simulink model "fullPlant"  (R2019a)
settings: Solver=VariableStepAuto  StartTime=0.0  StopTime=10.0  RelTol=1e-3
values from neighbouring files (symbols this model uses):
  alpha0 = 2    [aeroData.mat]
  b = 4.33    [aeroData.mat]
  c = 0.636    [aeroData.mat]
  CD = [0.01 0.012 0.015 0.019 0.024 0.03 0.036 0.044 0.052 0.01 0.012 0.015 ... (27 elements, 9x3)]    [aeroData.mat]
  Cl = [0.00012 -0.000325 -0.000768 -0.00121 -0.00165 -0.00209 -0.002529 -0.002968 -0.003408 -0.003849 -0.004292 0.002212 ... (33 elements, 11x3)]    [aeroData.mat]
  CL = [0.251 0.336 0.421 0.506 0.591 0.675 0.759 0.842 0.925 0.239 0.325 0.41 ... (27 elements, 9x3)]    [aeroData.mat]
  Clp = -0.00816971169566    [aeroData.mat]
  Clr = 0.00184411488766    [aeroData.mat]
  Cm = [-0.024 -0.038 -0.053 -0.068 -0.083 -0.098 -0.113 -0.128 -0.143 0.009 -0.005 -0.019 ... (27 elements, 9x3)]    [aeroData.mat]
  Cmq = -0.156184278773    [aeroData.mat]
  Cn = [-0.003061 -0.000518 0.002031 0.004586 0.007141 0.009696 0.012246 0.01479 0.017324 0.019845 0.022352 -0.012727 ... (33 elements, 11x3)]    [aeroData.mat]
  Cnp = -0.000739408737607    [aeroData.mat]
  Cnr = -0.00225688525575    [aeroData.mat]
  CY = [0.007395 0.001575 -0.004243 -0.010063 -0.015881 -0.021696 -0.027509 -0.033318 -0.039118 -0.044916 -0.050714 0.029115 ... (33 elements, 11x3)]    [aeroData.mat]
  g = 9.81    [aeroData.mat]
  gamma0 = -2.8361410859    [aeroData.mat]
  Ixx = 5.6481    [aeroData.mat]
  Iyy = 6.01051    [aeroData.mat]
  Izz = 11.4233    [aeroData.mat]
  m = 38    [aeroData.mat]
  S = 2.678    [aeroData.mat]
  V0 = 27    [aeroData.mat]
libraries: simulink x4, simulink_extras x3, aerolib6dof2 x1, aerolibatmos2 x1, aerolibasang x1, aerolibtransform2 x1, sharedtransform x1
settings Model: Creator=Admin  LastModifiedBy=Admin

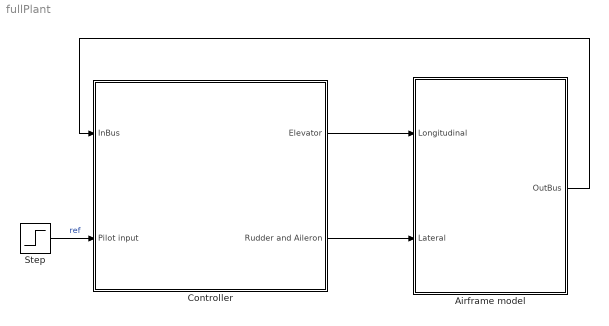
== system fullPlant ==
  Airframe model : Subsystem
  Controller : Subsystem
  Step : Step  Time=5  SampleTime=0
  wires:
  Step/1 -> Controller/2(Pilot input)  "ref"
  Controller/1(Elevator) -> Airframe model/1(Longitudinal)
  Controller/2(Rudder and Aileron) -> Airframe model/2(Lateral)
  Airframe model/1(OutBus) -> Controller/1(InBus)

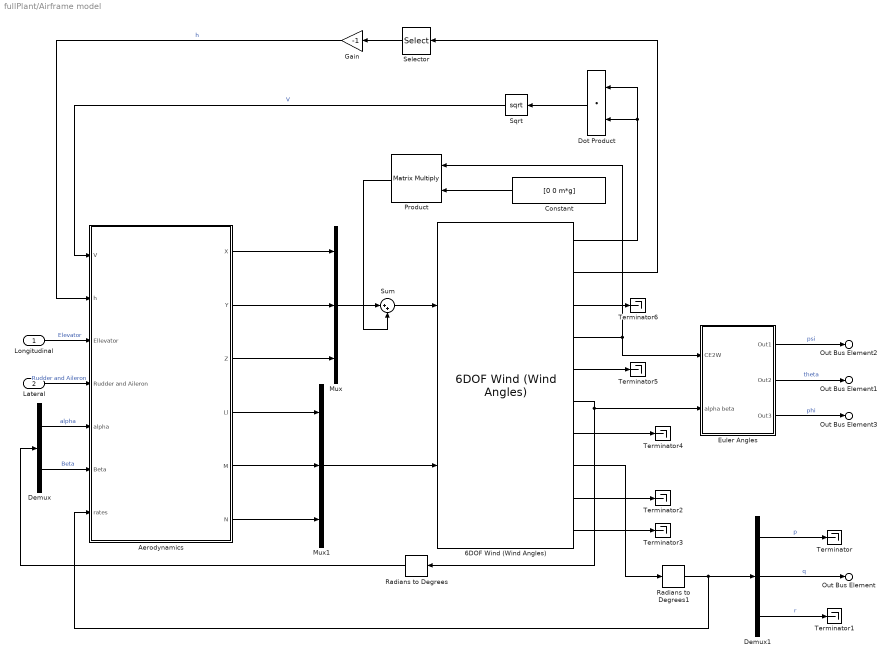
== system fullPlant/Airframe model ==
  Longitudinal : Inport
  Lateral : Inport  Port=2
  6DOF Wind (Wind Angles) : aerolib6dof2/6DOF Wind (Wind Angles)  units=Metric (MKS)  mtype=Fixed  rep=Wind Angles  xme_0=[0 0 -1000]  Vm_0=[V0 deg2rad(alpha0) 0]  wind_0=[0 deg2rad(gamma0) 0]  pm_0=[0 0 0]  mass_0=m  mass_e=0.5  mass_f=2.0  inertia=diag([Ixx Iyy Izz])  inertia_e=eye(3)  inertia_f=2*eye(3)  vre_flag=on  abi_flag=off  xme_statename=''  Vm_statename=''  alpha_statename=''  beta_statename=''  wind_statename=''  quat_statename=''  pm_statename=''  mass_statename=''
      settings: SourceProductName=Aerospace Blockset  SourceProductBaseCode=AE
  Aerodynamics : Subsystem
  Constant : Constant  Value=[0 0 m*g]
  Demux : Demux  Outputs=2
  Demux1 : Demux  Outputs=3
  Dot Product : DotProduct  InputSameDT=on  OutDataTypeStr=Inherit: Inherit via internal rule
  Euler Angles : Subsystem
  Gain : Gain  Gain=-1
  Mux : Mux  Inputs=3
  Mux1 : Mux  Inputs=3
  Product : Product  Multiplication=Matrix(*)
  Radians to Degrees : simulink_extras/Transformations/Radians to Degrees
  Radians to Degrees1 : simulink_extras/Transformations/Radians to Degrees
  Selector : Selector  InputPortWidth=3  IndexOptions=Index vector (dialog)  Indices=3  OutputSizes=1
  Sqrt : Sqrt  SaturateOnIntegerOverflow=on
  Sum : Sum  Inputs=|++
  Terminator{,1..6} (7 alike) : Terminator
  Out Bus Element : Outport  PortName=OutBus  Element=q
  Out Bus Element1 : Outport  PortName=OutBus  Element=theta
  Out Bus Element2 : Outport  PortName=OutBus  Element=psi
  Out Bus Element3 : Outport  PortName=OutBus  Element=phi
  wires:
  6DOF Wind (Wind Angles)/5 -> Terminator5/1
  Demux1/2 -> Out Bus Element/1  "q"
  Aerodynamics/4(Ll) -> Mux1/1
  Longitudinal/1 -> Aerodynamics/3(Ellevator)  "Elevator"
  Demux1/3 -> Terminator1/1  "r"
  6DOF Wind (Wind Angles)/4 -> Euler Angles/1(CE2W), Product/1
  Aerodynamics/5(M) -> Mux1/2
  6DOF Wind (Wind Angles)/9 -> Terminator2/1
  6DOF Wind (Wind Angles)/6 -> Radians to Degrees/1, Euler Angles/2(alpha beta)
  6DOF Wind (Wind Angles)/2 -> Selector/1
  6DOF Wind (Wind Angles)/10 -> Terminator3/1
  Lateral/1 -> Aerodynamics/4(Rudder and Aileron)  "Rudder and Aileron"
  Aerodynamics/3(Z) -> Mux/3
  Euler Angles/1(Out1) -> Out Bus Element2/1  "psi"
  6DOF Wind (Wind Angles)/1 -> Dot Product/1, Dot Product/2
  Aerodynamics/2(Y) -> Mux/2
  Demux/2 -> Aerodynamics/6(Beta)  "Beta"
  Sqrt/1 -> Aerodynamics/1(V)  "V"
  Dot Product/1 -> Sqrt/1
  Product/1 -> Sum/2
  6DOF Wind (Wind Angles)/3 -> Terminator6/1
  6DOF Wind (Wind Angles)/7 -> Terminator4/1
  Gain/1 -> Aerodynamics/2(h)  "h"
  Radians to Degrees/1 -> Demux/1
  Mux1/1 -> 6DOF Wind (Wind Angles)/2
  Aerodynamics/1(X) -> Mux/1
  Selector/1 -> Gain/1
  Euler Angles/3(Out3) -> Out Bus Element3/1  "phi"
  Euler Angles/2(Out2) -> Out Bus Element1/1  "theta"
  Mux/1 -> Sum/1
  Demux1/1 -> Terminator/1  "p"
  6DOF Wind (Wind Angles)/8 -> Radians to Degrees1/1
  Aerodynamics/6(N) -> Mux1/3
  Radians to Degrees1/1 -> Demux1/1, Aerodynamics/7(rates)
  Sum/1 -> 6DOF Wind (Wind Angles)/1
  Constant/1 -> Product/2
  Demux/1 -> Aerodynamics/5(alpha)  "alpha"

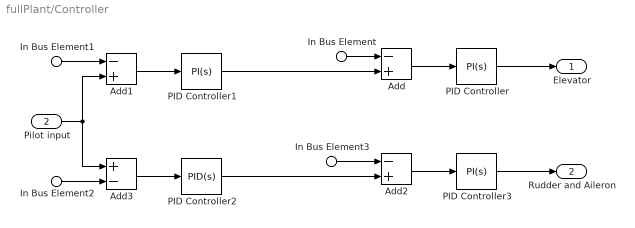
== system fullPlant/Controller ==
  In Bus Element : Inport  PortName=InBus  Element=q
  In Bus Element1 : Inport  PortName=InBus  Element=theta
  In Bus Element2 : Inport  PortName=InBus  Element=psi
  In Bus Element3 : Inport  PortName=InBus  Element=phi
  Pilot input : Inport  Port=2
  Add : Sum  Inputs=-+
  Add1 : Sum  Inputs=-+
  Add2 : Sum  Inputs=-+
  Add3 : Sum  Inputs=+-
  PID Controller : simulink/Continuous/PID Controller  Controller=PI  Form=Parallel  TimeDomain=Continuous-time  SampleTime=-1  IntegratorMethod=Forward Euler  FilterMethod=Forward Euler  ControllerParametersSource=internal  P=0.266196073930742  I=6.12743262101083  D=0  UseFilter=on  N=100  TunerSelectOption=Transfer Function Based (PID Tuner App)  InitialConditionSource=internal  InitialConditionForIntegrator=0  InitialConditionForFilter=0  DifferentiatorICPrevScaledInput=0  ExternalReset=none  TrackingMode=off  Kt=1  LimitOutput=off  UpperSaturationLimit=inf  LowerSaturationLimit=-inf  LinearizeAsGain=on  AntiWindupMode=none  Kb=1  POutMin=[]  POutMax=[]  IOutMin=[]  IOutMax=[]  DOutMin=[]  DOutMax=[]  NOutMin=[]  NOutMax=[]  SumOutMin=[]  SumOutMax=[]  SaturationOutMin=[]  SaturationOutMax=[]  PParamMin=[]  PParamMax=[]  IParamMin=[]  IParamMax=[]  DParamMin=[]  DParamMax=[]  NParamMin=[]  NParamMax=[]  KbParamMin=[]  KbParamMax=[]  KtParamMin=[]  KtParamMax=[]  KbOutMin=[]  KbOutMax=[]  KtOutMin=[]  KtOutMax=[]  IntegratorOutMin=[]  IntegratorOutMax=[]  FilterOutMin=[]  FilterOutMax=[]  SumI1OutMin=[]  SumI1OutMax=[]  SumI2OutMin=[]  SumI2OutMax=[]  SumI3OutMin=[]  SumI3OutMax=[]  SumI4OutMin=[]  SumI4OutMax=[]  SumDOutMin=[]  SumDOutMax=[]  DifferentiatorOutMin=[]  DifferentiatorOutMax=[]  FilterDiffOutCoefMin=[]  FilterDiffOutCoefMax=[]  ReciprocalOutMin=[]  ReciprocalOutMax=[]  SumDenOutMin=[]  SumDenOutMax=[]  SumNumOutMin=[]  SumNumOutMax=[]  DivideOutMin=[]  DivideOutMax=[]  IntegratorContinuousStateAttributes=''  IntegratorStateMustResolveToSignalObject=off  IntegratorRTWStateStorageClass=Auto  FilterContinuousStateAttributes=''  FilterStateMustResolveToSignalObject=off  FilterRTWStateStorageClass=Auto  ParallelPVariant=InternalParameters  IdealPVariant=Disabled  IVariant=InternalParameters  DVariant=Disabled  IntegratorVariant=Continuous  SatVariant=Disabled  AWVariant=Passthrough  PCopyVariant=Disabled  TRVariant=Disabled  FdbkBlocksVariant=Forward  IdealPFdbkVariant=Disabled  SatFdbkVariant=Disabled  DerivativeFilterVariant=Disabled  NVariant=Disabled  NCopyVariant=Disabled_SignalSpec  FilterICVariant=Disabled  IntegratorICVariant=InternalICs  ExternalResetVariant=Disabled  TRSumVariant=Passthrough  SumFdbkVariant=Disabled  SumVariant=Sum_PI
  PID Controller1 : simulink/Continuous/PID Controller  Controller=PI  Form=Parallel  TimeDomain=Continuous-time  SampleTime=-1  IntegratorMethod=Forward Euler  FilterMethod=Forward Euler  ControllerParametersSource=internal  P=45.6473930824707  I=259.27502213432  D=0  UseFilter=on  N=100  TunerSelectOption=Transfer Function Based (PID Tuner App)  InitialConditionSource=internal  InitialConditionForIntegrator=0  InitialConditionForFilter=0  DifferentiatorICPrevScaledInput=0  ExternalReset=none  TrackingMode=off  Kt=1  LimitOutput=off  UpperSaturationLimit=inf  LowerSaturationLimit=-inf  LinearizeAsGain=on  AntiWindupMode=none  Kb=1  POutMin=[]  POutMax=[]  IOutMin=[]  IOutMax=[]  DOutMin=[]  DOutMax=[]  NOutMin=[]  NOutMax=[]  SumOutMin=[]  SumOutMax=[]  SaturationOutMin=[]  SaturationOutMax=[]  PParamMin=[]  PParamMax=[]  IParamMin=[]  IParamMax=[]  DParamMin=[]  DParamMax=[]  NParamMin=[]  NParamMax=[]  KbParamMin=[]  KbParamMax=[]  KtParamMin=[]  KtParamMax=[]  KbOutMin=[]  KbOutMax=[]  KtOutMin=[]  KtOutMax=[]  IntegratorOutMin=[]  IntegratorOutMax=[]  FilterOutMin=[]  FilterOutMax=[]  SumI1OutMin=[]  SumI1OutMax=[]  SumI2OutMin=[]  SumI2OutMax=[]  SumI3OutMin=[]  SumI3OutMax=[]  SumI4OutMin=[]  SumI4OutMax=[]  SumDOutMin=[]  SumDOutMax=[]  DifferentiatorOutMin=[]  DifferentiatorOutMax=[]  FilterDiffOutCoefMin=[]  FilterDiffOutCoefMax=[]  ReciprocalOutMin=[]  ReciprocalOutMax=[]  SumDenOutMin=[]  SumDenOutMax=[]  SumNumOutMin=[]  SumNumOutMax=[]  DivideOutMin=[]  DivideOutMax=[]  IntegratorContinuousStateAttributes=''  IntegratorStateMustResolveToSignalObject=off  IntegratorRTWStateStorageClass=Auto  FilterContinuousStateAttributes=''  FilterStateMustResolveToSignalObject=off  FilterRTWStateStorageClass=Auto  ParallelPVariant=InternalParameters  IdealPVariant=Disabled  IVariant=InternalParameters  DVariant=Disabled  IntegratorVariant=Continuous  SatVariant=Disabled  AWVariant=Passthrough  PCopyVariant=Disabled  TRVariant=Disabled  FdbkBlocksVariant=Forward  IdealPFdbkVariant=Disabled  SatFdbkVariant=Disabled  DerivativeFilterVariant=Disabled  NVariant=Disabled  NCopyVariant=Disabled_SignalSpec  FilterICVariant=Disabled  IntegratorICVariant=InternalICs  ExternalResetVariant=Disabled  TRSumVariant=Passthrough  SumFdbkVariant=Disabled  SumVariant=Sum_PI
  PID Controller2 : simulink/Continuous/PID Controller  Controller=PID  Form=Parallel  TimeDomain=Continuous-time  SampleTime=-1  IntegratorMethod=Forward Euler  FilterMethod=Forward Euler  ControllerParametersSource=internal  P=-78.0232677726805  I=-57.2911628645873  D=-0.313797896413939  UseFilter=on  N=84.1674279209909  TunerSelectOption=Transfer Function Based (PID Tuner App)  InitialConditionSource=internal  InitialConditionForIntegrator=0  InitialConditionForFilter=0  DifferentiatorICPrevScaledInput=0  ExternalReset=none  TrackingMode=off  Kt=1  LimitOutput=off  UpperSaturationLimit=inf  LowerSaturationLimit=-inf  LinearizeAsGain=on  AntiWindupMode=none  Kb=1  POutMin=[]  POutMax=[]  IOutMin=[]  IOutMax=[]  DOutMin=[]  DOutMax=[]  NOutMin=[]  NOutMax=[]  SumOutMin=[]  SumOutMax=[]  SaturationOutMin=[]  SaturationOutMax=[]  PParamMin=[]  PParamMax=[]  IParamMin=[]  IParamMax=[]  DParamMin=[]  DParamMax=[]  NParamMin=[]  NParamMax=[]  KbParamMin=[]  KbParamMax=[]  KtParamMin=[]  KtParamMax=[]  KbOutMin=[]  KbOutMax=[]  KtOutMin=[]  KtOutMax=[]  IntegratorOutMin=[]  IntegratorOutMax=[]  FilterOutMin=[]  FilterOutMax=[]  SumI1OutMin=[]  SumI1OutMax=[]  SumI2OutMin=[]  SumI2OutMax=[]  SumI3OutMin=[]  SumI3OutMax=[]  SumI4OutMin=[]  SumI4OutMax=[]  SumDOutMin=[]  SumDOutMax=[]  DifferentiatorOutMin=[]  DifferentiatorOutMax=[]  FilterDiffOutCoefMin=[]  FilterDiffOutCoefMax=[]  ReciprocalOutMin=[]  ReciprocalOutMax=[]  SumDenOutMin=[]  SumDenOutMax=[]  SumNumOutMin=[]  SumNumOutMax=[]  DivideOutMin=[]  DivideOutMax=[]  IntegratorContinuousStateAttributes=''  IntegratorStateMustResolveToSignalObject=off  IntegratorRTWStateStorageClass=Auto  FilterContinuousStateAttributes=''  FilterStateMustResolveToSignalObject=off  FilterRTWStateStorageClass=Auto  ParallelPVariant=InternalParameters  IdealPVariant=Disabled  IVariant=InternalParameters  DVariant=InternalParameters  IntegratorVariant=Continuous  SatVariant=Disabled  AWVariant=Passthrough  PCopyVariant=Disabled  TRVariant=Disabled  FdbkBlocksVariant=Forward  IdealPFdbkVariant=Disabled  SatFdbkVariant=Disabled  DerivativeFilterVariant=ContFilter  NVariant=InternalParameters  NCopyVariant=Disabled  FilterICVariant=InternalICsFilter  IntegratorICVariant=InternalICs  ExternalResetVariant=Disabled  TRSumVariant=Passthrough  SumFdbkVariant=Disabled  SumVariant=Sum_PID
  PID Controller3 : simulink/Continuous/PID Controller  Controller=PI  Form=Parallel  TimeDomain=Continuous-time  SampleTime=-1  IntegratorMethod=Forward Euler  FilterMethod=Forward Euler  ControllerParametersSource=internal  P=0.0847633233542449  I=0.0359518424251433  D=0  UseFilter=on  N=100  TunerSelectOption=Transfer Function Based (PID Tuner App)  InitialConditionSource=internal  InitialConditionForIntegrator=0  InitialConditionForFilter=0  DifferentiatorICPrevScaledInput=0  ExternalReset=none  TrackingMode=off  Kt=1  LimitOutput=off  UpperSaturationLimit=inf  LowerSaturationLimit=-inf  LinearizeAsGain=on  AntiWindupMode=none  Kb=1  POutMin=[]  POutMax=[]  IOutMin=[]  IOutMax=[]  DOutMin=[]  DOutMax=[]  NOutMin=[]  NOutMax=[]  SumOutMin=[]  SumOutMax=[]  SaturationOutMin=[]  SaturationOutMax=[]  PParamMin=[]  PParamMax=[]  IParamMin=[]  IParamMax=[]  DParamMin=[]  DParamMax=[]  NParamMin=[]  NParamMax=[]  KbParamMin=[]  KbParamMax=[]  KtParamMin=[]  KtParamMax=[]  KbOutMin=[]  KbOutMax=[]  KtOutMin=[]  KtOutMax=[]  IntegratorOutMin=[]  IntegratorOutMax=[]  FilterOutMin=[]  FilterOutMax=[]  SumI1OutMin=[]  SumI1OutMax=[]  SumI2OutMin=[]  SumI2OutMax=[]  SumI3OutMin=[]  SumI3OutMax=[]  SumI4OutMin=[]  SumI4OutMax=[]  SumDOutMin=[]  SumDOutMax=[]  DifferentiatorOutMin=[]  DifferentiatorOutMax=[]  FilterDiffOutCoefMin=[]  FilterDiffOutCoefMax=[]  ReciprocalOutMin=[]  ReciprocalOutMax=[]  SumDenOutMin=[]  SumDenOutMax=[]  SumNumOutMin=[]  SumNumOutMax=[]  DivideOutMin=[]  DivideOutMax=[]  IntegratorContinuousStateAttributes=''  IntegratorStateMustResolveToSignalObject=off  IntegratorRTWStateStorageClass=Auto  FilterContinuousStateAttributes=''  FilterStateMustResolveToSignalObject=off  FilterRTWStateStorageClass=Auto  ParallelPVariant=InternalParameters  IdealPVariant=Disabled  IVariant=InternalParameters  DVariant=Disabled  IntegratorVariant=Continuous  SatVariant=Disabled  AWVariant=Passthrough  PCopyVariant=Disabled  TRVariant=Disabled  FdbkBlocksVariant=Forward  IdealPFdbkVariant=Disabled  SatFdbkVariant=Disabled  DerivativeFilterVariant=Disabled  NVariant=Disabled  NCopyVariant=Disabled_SignalSpec  FilterICVariant=Disabled  IntegratorICVariant=InternalICs  ExternalResetVariant=Disabled  TRSumVariant=Passthrough  SumFdbkVariant=Disabled  SumVariant=Sum_PI
  Elevator : Outport
  Rudder and Aileron : Outport  Port=2
  wires:
  PID Controller2/1 -> Add2/2
  Add1/1 -> PID Controller1/1
  Pilot input/1 -> Add1/2, Add3/1
  Add3/1 -> PID Controller2/1
  Add2/1 -> PID Controller3/1
  Add/1 -> PID Controller/1
  PID Controller3/1 -> Rudder and Aileron/1
  PID Controller1/1 -> Add/2
  In Bus Element3/1 -> Add2/1
  In Bus Element2/1 -> Add3/2
  In Bus Element/1 -> Add/1
  In Bus Element1/1 -> Add1/1
  PID Controller/1 -> Elevator/1

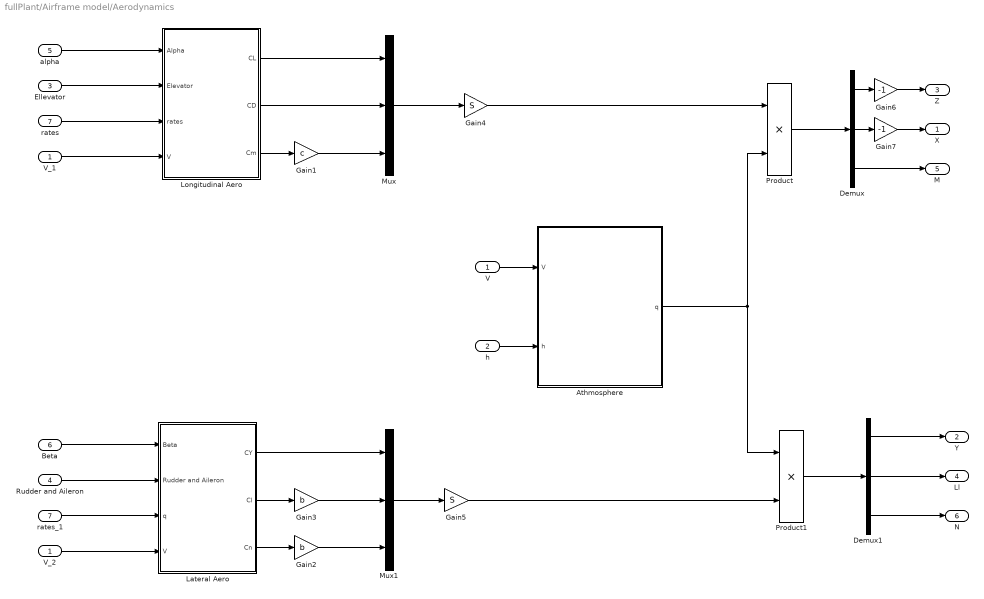
== system fullPlant/Airframe model/Aerodynamics ==
  V : Inport
  h : Inport  Port=2
  Ellevator : Inport  Port=3
  Rudder and Aileron : Inport  Port=4
  alpha : Inport  Port=5
  Beta : Inport  Port=6
  rates : Inport  Port=7
  Athmosphere : Subsystem
  Demux : Demux  Outputs=3
  Demux1 : Demux  Outputs=3
  Gain1 : Gain  Gain=c
  Gain2 : Gain  Gain=b
  Gain3 : Gain  Gain=b
  Gain4 : Gain  Gain=S
  Gain5 : Gain  Gain=S
  Gain6 : Gain  Gain=-1
  Gain7 : Gain  Gain=-1
  Lateral Aero : Subsystem
  "Longitudinal Aero " : Subsystem
  Mux : Mux  Inputs=3
  Mux1 : Mux  Inputs=3
  Product : Product
  Product1 : Product
  V_1 : InportShadow
  V_2 : InportShadow
  rates_1 : InportShadow  Port=7
  X : Outport
  Y : Outport  Port=2
  Z : Outport  Port=3
  Ll : Outport  Port=4
  M : Outport  Port=5
  N : Outport  Port=6
  wires:
  "Longitudinal Aero "/3(Cm) -> Gain1/1
  rates_1/1 -> Lateral Aero/3(q)
  Demux/2 -> Gain7/1
  Lateral Aero/1(CY) -> Mux1/1
  V_2/1 -> Lateral Aero/4("V ")
  Gain1/1 -> Mux/3
  Ellevator/1 -> "Longitudinal Aero "/2(Elevator)
  Gain3/1 -> Mux1/2
  V_1/1 -> "Longitudinal Aero "/4("V ")
  rates/1 -> "Longitudinal Aero "/3(rates)
  Mux1/1 -> Gain5/1
  Demux1/1 -> Y/1
  Gain4/1 -> Product/1
  Gain5/1 -> Product1/2
  Demux/1 -> Gain6/1
  alpha/1 -> "Longitudinal Aero "/1(Alpha)
  Rudder and Aileron/1 -> Lateral Aero/2(Rudder and Aileron)
  Beta/1 -> Lateral Aero/1(Beta)
  Gain2/1 -> Mux1/3
  Demux/3 -> M/1
  Gain6/1 -> Z/1
  "Longitudinal Aero "/1(CL) -> Mux/1
  "Longitudinal Aero "/2(CD) -> Mux/2
  Mux/1 -> Gain4/1
  Product1/1 -> Demux1/1
  Product/1 -> Demux/1
  Lateral Aero/3(Cn) -> Gain2/1
  Lateral Aero/2(Cl) -> Gain3/1
  Demux1/3 -> N/1
  Demux1/2 -> Ll/1
  Gain7/1 -> X/1
  Athmosphere/1(q) -> Product1/1, Product/2
  V/1 -> Athmosphere/1(V)
  h/1 -> Athmosphere/2(h)

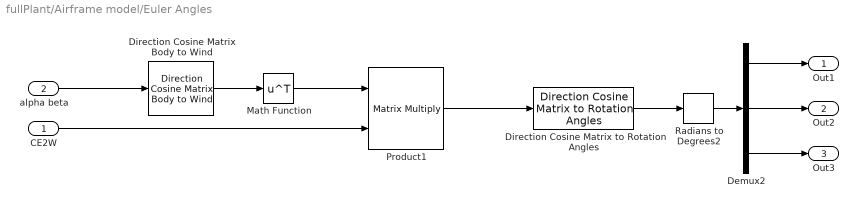
== system fullPlant/Airframe model/Euler Angles ==
  CE2W : Inport
  alpha beta : Inport  Port=2
  Demux2 : Demux  Outputs=3
  Direction Cosine Matrix Body to Wind : aerolibtransform2/Direction Cosine Matrix Body to Wind
      settings: SourceProductName=Aerospace Blockset  SourceProductBaseCode=AE
  Direction Cosine Matrix to Rotation Angles : sharedtransform/Direction Cosine Matrix to Rotation Angles  rotationOrder=ZYX  aMode=aMode  action=None  tolerance=eps(2)
      settings: SourceProductName=Aerospace Blockset  SourceProductBaseCode=AE
  Math Function : Math  Operator=transpose  SaturateOnIntegerOverflow=on
  Product1 : Product  Multiplication=Matrix(*)
  Radians to Degrees2 : simulink_extras/Transformations/Radians to Degrees
  Out1 : Outport
  Out2 : Outport  Port=2
  Out3 : Outport  Port=3
  wires:
  Demux2/3 -> Out3/1
  alpha beta/1 -> Direction Cosine Matrix Body to Wind/1
  Product1/1 -> Direction Cosine Matrix to Rotation Angles/1
  Demux2/1 -> Out1/1
  Math Function/1 -> Product1/1
  Direction Cosine Matrix to Rotation Angles/1 -> Radians to Degrees2/1
  Demux2/2 -> Out2/1
  CE2W/1 -> Product1/2
  Radians to Degrees2/1 -> Demux2/1
  Direction Cosine Matrix Body to Wind/1 -> Math Function/1

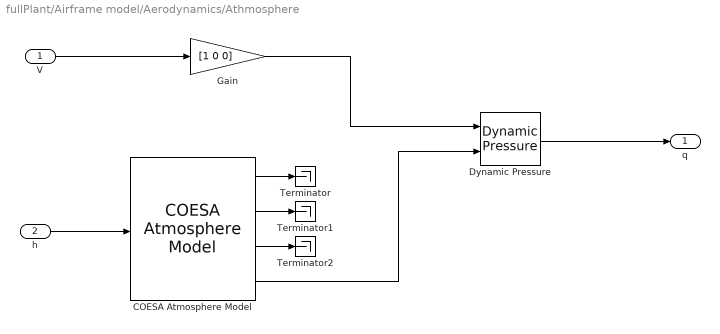
== system fullPlant/Airframe model/Aerodynamics/Athmosphere ==
  V : Inport
  h : Inport  Port=2
  COESA Atmosphere Model : aerolibatmos2/COESA Atmosphere Model  units=Metric (MKS)  spec=1976 COESA-extended U.S. Standard Atmosphere  model=Profile  profile_var=High temperature  profile_percent=1%  profile_alt=5 km (16404 ft)  envelope_var=High temperature  envelope_percent=1%  action=Warning
  Dynamic Pressure : aerolibasang/Dynamic Pressure
  Gain : Gain  Gain=[1 0 0]
  Terminator : Terminator
  Terminator1 : Terminator
  Terminator2 : Terminator
  q : Outport
  wires:
  COESA Atmosphere Model/2 -> Terminator1/1
  Gain/1 -> Dynamic Pressure/1
  COESA Atmosphere Model/1 -> Terminator/1
  COESA Atmosphere Model/3 -> Terminator2/1
  Dynamic Pressure/1 -> q/1
  h/1 -> COESA Atmosphere Model/1
  V/1 -> Gain/1
  COESA Atmosphere Model/4 -> Dynamic Pressure/2

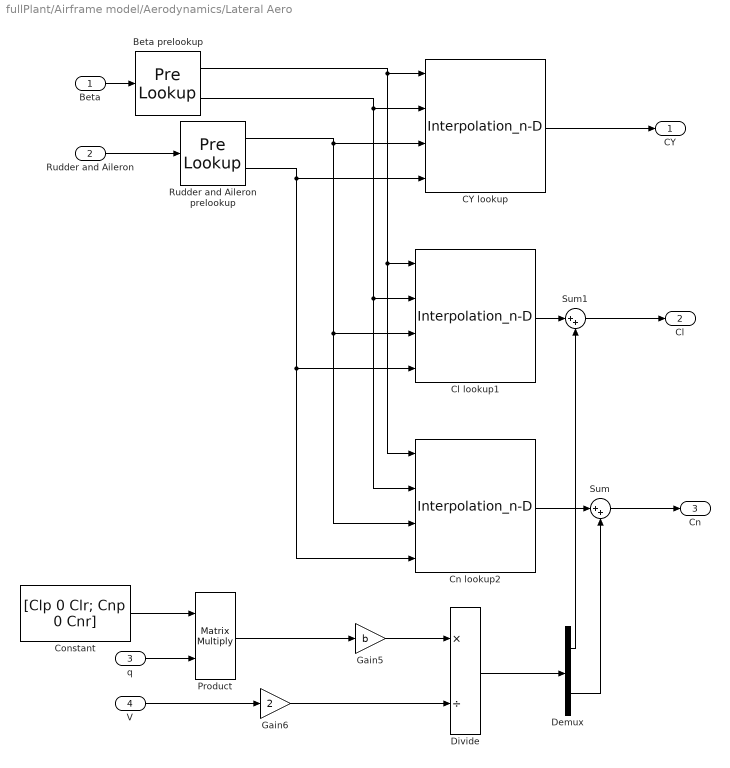
== system fullPlant/Airframe model/Aerodynamics/Lateral Aero ==
  Beta : Inport
  Rudder and Aileron : Inport  Port=2
  q : Inport  Port=3  PortDimensions=3
  "V " : Inport  Port=4
  "Beta prelookup " : PreLookup  BreakpointsData=Beta  ExtrapMethod=Linear
  CY lookup : Interpolation_n-D  Table=CY  InternalRulePriority=Speed
  Cl lookup1 : Interpolation_n-D  Table=Cl  InternalRulePriority=Speed
  Cn lookup2 : Interpolation_n-D  Table=Cn  InternalRulePriority=Speed
  Constant : Constant  Value=[Clp 0 Clr; Cnp 0 Cnr]
  Demux : Demux  Outputs=2
  Divide : Product  Inputs=*/
  Gain5 : Gain  Gain=b
  Gain6 : Gain  Gain=2
  Product : Product  Multiplication=Matrix(*)
  Rudder and Aileron prelookup : PreLookup  BreakpointsData=Rudder  ExtrapMethod=Linear
  Sum : Sum  Inputs=|++
  Sum1 : Sum  Inputs=|++
  CY : Outport
  Cl : Outport  Port=2
  Cn : Outport  Port=3
  wires:
  CY lookup/1 -> CY/1
  Product/1 -> Gain5/1
  "V "/1 -> Gain6/1
  Gain6/1 -> Divide/2
  Gain5/1 -> Divide/1
  Cn lookup2/1 -> Sum/1
  Sum/1 -> Cn/1
  Rudder and Aileron/1 -> Rudder and Aileron prelookup/1
  Beta/1 -> "Beta prelookup "/1
  "Beta prelookup "/2 -> CY lookup/2, Cl lookup1/2, Cn lookup2/2
  Rudder and Aileron prelookup/1 -> CY lookup/3, Cl lookup1/3, Cn lookup2/3
  "Beta prelookup "/1 -> CY lookup/1, Cl lookup1/1, Cn lookup2/1
  Rudder and Aileron prelookup/2 -> CY lookup/4, Cl lookup1/4, Cn lookup2/4
  Cl lookup1/1 -> Sum1/1
  Sum1/1 -> Cl/1
  q/1 -> Product/2
  Constant/1 -> Product/1
  Divide/1 -> Demux/1
  Demux/1 -> Sum1/2
  Demux/2 -> Sum/2

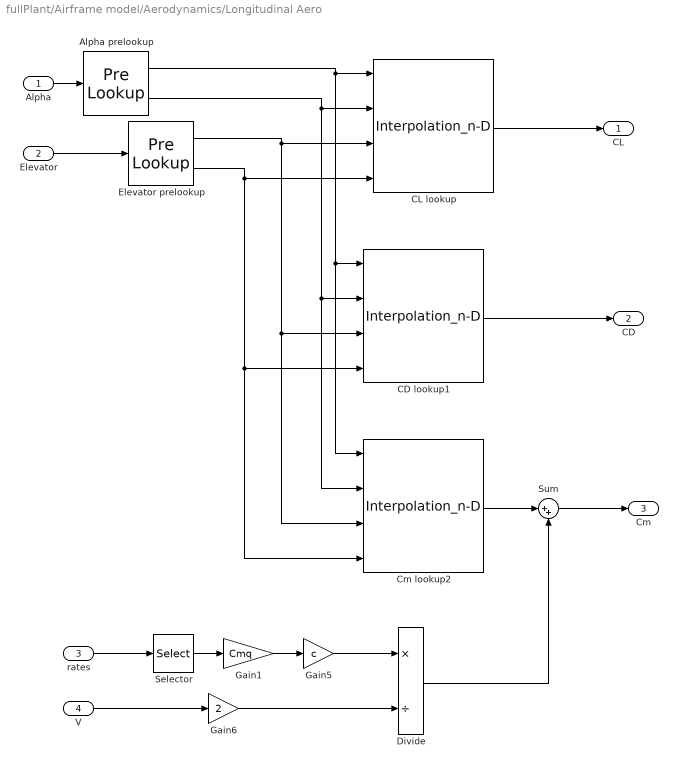
== system fullPlant/Airframe model/Aerodynamics/Longitudinal Aero  ==
  Alpha : Inport
  Elevator : Inport  Port=2
  rates : Inport  Port=3
  "V " : Inport  Port=4
  "Alpha prelookup " : PreLookup  BreakpointsData=alpha  ExtrapMethod=Linear
  CD lookup1 : Interpolation_n-D  Table=CD  InternalRulePriority=Speed
  CL lookup : Interpolation_n-D  Table=CL  InternalRulePriority=Speed
  Cm lookup2 : Interpolation_n-D  Table=Cm  InternalRulePriority=Speed
  Divide : Product  Inputs=*/
  Elevator prelookup : PreLookup  BreakpointsData=Elevator  ExtrapMethod=Linear
  Gain1 : Gain  Gain=Cmq
  Gain5 : Gain  Gain=c
  Gain6 : Gain  Gain=2
  Selector : Selector  InputPortWidth=3  IndexOptions=Index vector (dialog)  Indices=2  OutputSizes=1
  Sum : Sum  Inputs=|++
  CL : Outport
  CD : Outport  Port=2
  Cm : Outport  Port=3
  wires:
  Elevator prelookup/2 -> Cm lookup2/4, CD lookup1/4, CL lookup/4
  "Alpha prelookup "/1 -> Cm lookup2/1, CD lookup1/1, CL lookup/1
  Elevator prelookup/1 -> Cm lookup2/3, CD lookup1/3, CL lookup/3
  "Alpha prelookup "/2 -> Cm lookup2/2, CD lookup1/2, CL lookup/2
  Alpha/1 -> "Alpha prelookup "/1
  Elevator/1 -> Elevator prelookup/1
  Sum/1 -> Cm/1
  Cm lookup2/1 -> Sum/1
  Gain5/1 -> Divide/1
  Gain6/1 -> Divide/2
  rates/1 -> Selector/1
  "V "/1 -> Gain6/1
  Divide/1 -> Sum/2
  Gain1/1 -> Gain5/1
  Selector/1 -> Gain1/1
  CD lookup1/1 -> CD/1
  CL lookup/1 -> CL/1
